simulink model "ES102A_PolarityCfg"  (R2013b)
settings: Solver=ode45  StartTime=0.0  StopTime=10.0  RelTol=1e-3
undefined symbols (not defined in the file): sigbuilder_block
libraries: simulink x29
(part 1 of 4)
settings Model: RequirementInfo={'doors' '00006113' '1' 'false' 'DOORS Surrogate Item' '' } %GIDa_8876c5aa_43e1_47bf_bb90_3f74317f85a0  reqMgrSettings="100 S'doors','misc'{{S'surrogatepath','savemodel','savesurrogate','updateLinks','doorsLinks2sl','slLinks2Doors','purgeDoors','purgeSimulink','detaillevel','surrogateId','synctime'{{T\"/ESG Group/ES102A_PolarityCfg\",M[1],M[1],M[0],M[0],M[0],M[0],M[0],M[1],T\"00006113\",T\"\"}},S'mode','pathStorage'{{T\"generic\",T\"modelRelative\"}}}}"  Creator=pz79n7  LastModifiedBy=NZG49T
settings DataIOCC: SaveFormat=Structure

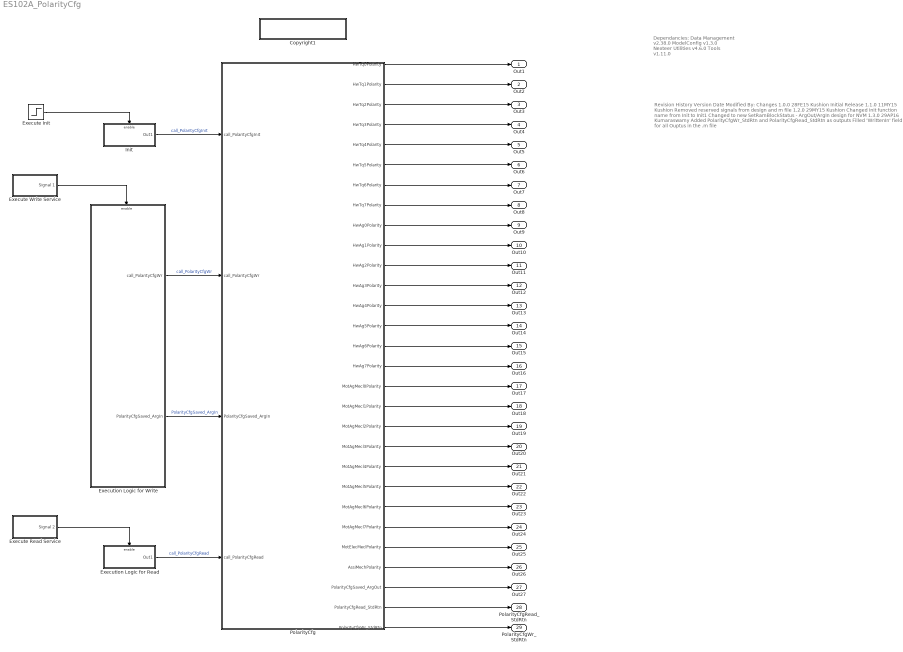
== system ES102A_PolarityCfg ==
  note: Revision History
      |
      | Version		Date 		Modified By: 		Changes
      | 1.0.0 		28FE15		Kushion			Initial Release
      | 1.1.0		11MY15		Kushion			Removed reserved signals from design and m file
      | 1.2.0              29MY15        Kushion			Changed init function name from Init to Init1
      | 										Changed to new SetRamBlockStatus - ArgOut/ArgIn design for NVM
      | 1.3.0		29AP16		Kumaraswamy	Added PolarityCfgWr_StdRtn and PolarityCfgRead_StdRtn as outputs
      | 										Filled 'WrittenIn' field for all Ouptus in the .m file
  note: Dependancies:
      |
      |    Data Management v2.38.0
      |    ModelConfig v1.3.0
      |    Nexteer Utilities v4.6.0
      |    Tools v1.11.0
  Copyright1 : Subsystem  Description=|  mask(Copyright Information){none=on}
      | Copyright info block.                                               
      |                                                                     
      | Place copyright information at the top of every subsystem in design.
      mask prompts: none "No parameters"
      mask help: Place copyright information at the top of every subsystem in design.
      mask Display:
      | NxtrConf = 'Nexteer Confidential';
      | 
      | sys = bdroot; %handle for the current model ("system")
      | first = get_param(sys,'Created');
      | if(isempty(first))
      |     first = datestr(now,'yyyy');
      | else
      |     first = first(end-3:end);  %year is last four digits
      | end
      | 
      | last = get_param(sys,'LastModifiedDate');
      | if isempty(last)
      |     last = datestr(now,'yyyy');
      | else
      |     last = last(end-3:end);
      | end
      | 
      | if strcmp(first,last)
      |     fprintf('%s\nCopyright  %s Nexteer',NxtrConf,first);
      | else
      |     fprintf('%s\n%s%s-%s Nexteer',NxtrConf,char(169),first,last);
      | end
  Execute Init : Step  Time=0.002  Before=1  After=0  SampleTime=0
  Execute Read Service : Subsystem  Tag=STV Subsys  RequirementInfo={} %GIDa_aa5db022_3107_4021_b4bb_b6752dc48d57  LoadFcn=sigbuilder_block('load');  StartFcn=sigbuilder_block('start');  StopFcn=sigbuilder_block('stop');  ClipboardFcn=sigbuilder_block('clipboard');  mask(Sigbuilder block){}
      mask help: Simulink:masks:SigbuilderBlock_MD
      mask init:
      | if ~strcmp(get_param(bdroot(gcbh),'SimulationStatus'),'stopped') tuvar = sigbuilder_block('maskInit'); end
      settings: CopyFcn=sigbuilder_block('copy');  DeleteFcn=sigbuilder_block('delete');  ModelCloseFcn=sigbuilder_block('modelClose');  PreSaveFcn=sigbuilder_block('preSave');  PauseFcn=sigbuilder_block('pause');  ContinueFcn=sigbuilder_block('continue');  NameChangeFcn=sigbuilder_block('namechange');  OpenFcn=sigbuilder_block('open',[437.25 118.5 550.5 394.5 ]);  CloseFcn=sigbuilder_block('close');
      mask Display: plot(0, 0, 100, 100,[2, 2, 32, 32, 2], [68, 8, 8, 68, 68],[32, 2], [38, 38], [32, 19, 2],[53, 60, 44], [32, 17, 17, 2],[16, 16, 31, 31]);txt = getActiveGroup(gcbh);text(2, 100, txt,'verticalAlignment', 'top');
  Execute Write Service : Subsystem  Tag=STV Subsys  RequirementInfo={} %GIDa_7764aa85_78e4_46ff_b91e_6bc780200c88  LoadFcn=sigbuilder_block('load');  StartFcn=sigbuilder_block('start');  StopFcn=sigbuilder_block('stop');  ClipboardFcn=sigbuilder_block('clipboard');  mask(Sigbuilder block){}
      mask help: Simulink:masks:SigbuilderBlock_MD
      mask init:
      | if ~strcmp(get_param(bdroot(gcbh),'SimulationStatus'),'stopped') tuvar = sigbuilder_block('maskInit'); end
      settings: CopyFcn=sigbuilder_block('copy');  DeleteFcn=sigbuilder_block('delete');  ModelCloseFcn=sigbuilder_block('modelClose');  PreSaveFcn=sigbuilder_block('preSave');  PauseFcn=sigbuilder_block('pause');  ContinueFcn=sigbuilder_block('continue');  NameChangeFcn=sigbuilder_block('namechange');  OpenFcn=sigbuilder_block('open',[437.25 118.5 550.5 394.5 ]);  CloseFcn=sigbuilder_block('close');
      mask Display: plot(0, 0, 100, 100,[2, 2, 32, 32, 2], [68, 8, 8, 68, 68],[32, 2], [38, 38], [32, 19, 2],[53, 60, 44], [32, 17, 17, 2],[16, 16, 31, 31]);txt = getActiveGroup(gcbh);text(2, 100, txt,'verticalAlignment', 'top');
  Execution Logic for Read : Subsystem  TreatAsAtomicUnit=on
  Execution Logic for Write : Subsystem  TreatAsAtomicUnit=on
  Init : Subsystem  TreatAsAtomicUnit=on
  PolarityCfg : Subsystem  RequirementInfo={'doors' '00006113' '2' 'false' 'DOORS Surrogate Item' '' } %GIDa_b5b2a4cf_7b68_4330_844c_0f051cc88fcd
      settings: AttributesFormatString=ES102A
  Out1 : Outport
  Out2 : Outport  Port=2
  Out3 : Outport  Port=3
  Out4 : Outport  Port=4
  Out5 : Outport  Port=5
  Out6 : Outport  Port=6
  Out7 : Outport  Port=7
  Out8 : Outport  Port=8
  Out9 : Outport  Port=9
  Out10 : Outport  Port=10
  Out11 : Outport  Port=11
  Out12 : Outport  Port=12
  Out13 : Outport  Port=13
  Out14 : Outport  Port=14
  Out15 : Outport  Port=15
  Out16 : Outport  Port=16
  Out17 : Outport  Port=17
  Out18 : Outport  Port=18
  Out19 : Outport  Port=19
  Out20 : Outport  Port=20
  Out21 : Outport  Port=21
  Out22 : Outport  Port=22
  Out23 : Outport  Port=23
  Out24 : Outport  Port=24
  Out25 : Outport  Port=25
  Out26 : Outport  Port=26
  Out27 : Outport  Port=27
  PolarityCfgRead_StdRtn : Outport  Port=28
  PolarityCfgWr_StdRtn : Outport  Port=29
  wires:
  Init/1(Out1) -> PolarityCfg/1(call_PolarityCfgInit)  "call_PolarityCfgInit"
  Execution Logic for Write/1(call_PolarityCfgWr) -> PolarityCfg/2(call_PolarityCfgWr)  "call_PolarityCfgWr"
  Execute Write Service/1(Signal 1) -> Execution Logic for Write/Enable
  PolarityCfg/1(HwTq0Polarity) -> Out1/1
  PolarityCfg/2(HwTq1Polarity) -> Out2/1
  PolarityCfg/3(HwTq2Polarity) -> Out3/1
  PolarityCfg/4(HwTq3Polarity) -> Out4/1
  PolarityCfg/5(HwTq4Polarity) -> Out5/1
  PolarityCfg/6(HwTq5Polarity) -> Out6/1
  PolarityCfg/7(HwTq6Polarity) -> Out7/1
  PolarityCfg/8(HwTq7Polarity) -> Out8/1
  PolarityCfg/9(HwAg0Polarity) -> Out9/1
  PolarityCfg/10(HwAg1Polarity) -> Out10/1
  PolarityCfg/11(HwAg2Polarity) -> Out11/1
  PolarityCfg/12(HwAg3Polarity) -> Out12/1
  PolarityCfg/13(HwAg4Polarity) -> Out13/1
  PolarityCfg/14(HwAg5Polarity) -> Out14/1
  PolarityCfg/15(HwAg6Polarity) -> Out15/1
  PolarityCfg/16(HwAg7Polarity) -> Out16/1
  PolarityCfg/17(MotAgMecl0Polarity) -> Out17/1
  PolarityCfg/18(MotAgMecl1Polarity) -> Out18/1
  PolarityCfg/19(MotAgMecl2Polarity) -> Out19/1
  PolarityCfg/20(MotAgMecl3Polarity) -> Out20/1
  PolarityCfg/21(MotAgMecl4Polarity) -> Out21/1
  PolarityCfg/22(MotAgMecl5Polarity) -> Out22/1
  PolarityCfg/23(MotAgMecl6Polarity) -> Out23/1
  PolarityCfg/24(MotAgMecl7Polarity) -> Out24/1
  PolarityCfg/25(MotElecMeclPolarity) -> Out25/1
  PolarityCfg/26(AssiMechPolarity) -> Out26/1
  Execute Init/1 -> Init/Enable
  Execution Logic for Read/1(Out1) -> PolarityCfg/4(call_PolarityCfgRead)  "call_PolarityCfgRead"
  Execute Read Service/1(Signal 2) -> Execution Logic for Read/Enable
  Execution Logic for Write/2(PolarityCfgSaved_ArgIn) -> PolarityCfg/3(PolarityCfgSaved_ArgIn)  "PolarityCfgSaved_ArgIn"
  PolarityCfg/27(PolarityCfgSaved_ArgOut) -> Out27/1
  PolarityCfg/29(PolarityCfgWr_StdRtn) -> PolarityCfgWr_StdRtn/1
  PolarityCfg/28(PolarityCfgRead_StdRtn) -> PolarityCfgRead_StdRtn/1

== system ES102A_PolarityCfg/Copyright1 ==

== system ES102A_PolarityCfg/Execute Read Service ==
  Demux : Demux  Tag=STV Demux  Outputs=1
  FromWs : FromWorkspace  Tag=STV FromWs  VariableName=tuvar  SampleTime=0
      SigBuilderData=|
      | common.afterFinalStr = 'Extrapolate'
      | common.sampleTime = 0
      | dataSet.timeRange = [0 10]
      | dataSet.name = 'Group 1'
      | sbobj.Groups.Name = 'Group 1'
      | sbobj.Groups.Signals.Name = 'Signal 2'
      | sbobj.Groups.Signals.XData = [0 5.02 5.02 5.3 5.3 10]
      | sbobj.Groups.Signals.YData = [0 0 1 1 0 0]
  Signal 2 : Outport  Tag=STV Outport
  wires:
  FromWs/1 -> Demux/1
  Demux/1 -> Signal 2/1

== system ES102A_PolarityCfg/Execute Write Service ==
  Demux : Demux  Tag=STV Demux  Outputs=1
  FromWs : FromWorkspace  Tag=STV FromWs  VariableName=tuvar  SampleTime=0
      SigBuilderData=|
      | common.afterFinalStr = 'Extrapolate'
      | common.sampleTime = 0
      | dataSet.timeRange = [0 10]
      | dataSet.name = 'Group 1'
      | sbobj.Groups.Name = 'Group 1'
      | sbobj.Groups.Signals.Name = 'Signal 1'
      | sbobj.Groups.Signals.XData = [0 2.02 2.02 2.12 2.12 10]
      | sbobj.Groups.Signals.YData = [0 0 1 1 0 0]
  Signal 1 : Outport  Tag=STV Outport
  wires:
  Demux/1 -> Signal 1/1
  FromWs/1 -> Demux/1

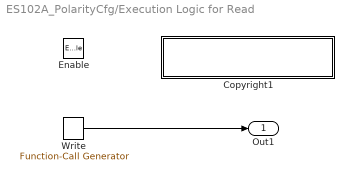
== system ES102A_PolarityCfg/Execution Logic for Read ==
  Enable : EnablePort
  Copyright1 : Subsystem  Description=|  mask(Copyright Information){none=on}
      | Copyright info block.                                               
      |                                                                     
      | Place copyright information at the top of every subsystem in design.
      mask prompts: none "No parameters"
      mask help: Place copyright information at the top of every subsystem in design.
      mask Display:
      | NxtrConf = 'Nexteer Confidential';
      | 
      | sys = bdroot; %handle for the current model ("system")
      | first = get_param(sys,'Created');
      | if(isempty(first))
      |     first = datestr(now,'yyyy');
      | else
      |     first = first(end-3:end);  %year is last four digits
      | end
      | 
      | last = get_param(sys,'LastModifiedDate');
      | if isempty(last)
      |     last = datestr(now,'yyyy');
      | else
      |     last = last(end-3:end);
      | end
      | 
      | if strcmp(first,last)
      |     fprintf('%s\nCopyright  %s Nexteer',NxtrConf,first);
      | else
      |     fprintf('%s\n%s%s-%s Nexteer',NxtrConf,char(169),first,last);
      | end
  "Write " : simulink/Ports & Subsystems/Function-Call Generator  sample_time=0.001  numberOfIterations=1
  Out1 : Outport
  wires:
  "Write "/1 -> Out1/1

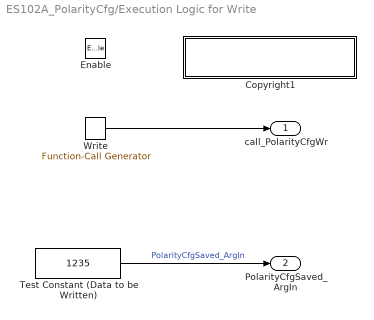
== system ES102A_PolarityCfg/Execution Logic for Write ==
  Enable : EnablePort
  Copyright1 : Subsystem  Description=|  mask(Copyright Information){none=on}
      | Copyright info block.                                               
      |                                                                     
      | Place copyright information at the top of every subsystem in design.
      mask prompts: none "No parameters"
      mask help: Place copyright information at the top of every subsystem in design.
      mask Display:
      | NxtrConf = 'Nexteer Confidential';
      | 
      | sys = bdroot; %handle for the current model ("system")
      | first = get_param(sys,'Created');
      | if(isempty(first))
      |     first = datestr(now,'yyyy');
      | else
      |     first = first(end-3:end);  %year is last four digits
      | end
      | 
      | last = get_param(sys,'LastModifiedDate');
      | if isempty(last)
      |     last = datestr(now,'yyyy');
      | else
      |     last = last(end-3:end);
      | end
      | 
      | if strcmp(first,last)
      |     fprintf('%s\nCopyright  %s Nexteer',NxtrConf,first);
      | else
      |     fprintf('%s\n%s%s-%s Nexteer',NxtrConf,char(169),first,last);
      | end
  Test Constant (Data to be Written) : Constant  Value=1235  OutDataTypeStr=uint32
  "Write " : simulink/Ports & Subsystems/Function-Call Generator  sample_time=0.001  numberOfIterations=1
  call_PolarityCfgWr : Outport
  PolarityCfgSaved_ArgIn : Outport  Port=2
  wires:
  "Write "/1 -> call_PolarityCfgWr/1
  Test Constant (Data to be Written)/1 -> PolarityCfgSaved_ArgIn/1  "PolarityCfgSaved_ArgIn"

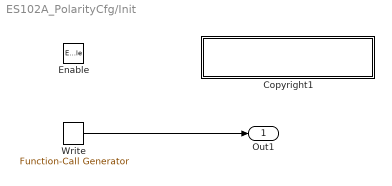
== system ES102A_PolarityCfg/Init ==
  Enable : EnablePort
  Copyright1 : Subsystem  Description=|  mask(Copyright Information){none=on}
      | Copyright info block.                                               
      |                                                                     
      | Place copyright information at the top of every subsystem in design.
      mask prompts: none "No parameters"
      mask help: Place copyright information at the top of every subsystem in design.
      mask Display:
      | NxtrConf = 'Nexteer Confidential';
      | 
      | sys = bdroot; %handle for the current model ("system")
      | first = get_param(sys,'Created');
      | if(isempty(first))
      |     first = datestr(now,'yyyy');
      | else
      |     first = first(end-3:end);  %year is last four digits
      | end
      | 
      | last = get_param(sys,'LastModifiedDate');
      | if isempty(last)
      |     last = datestr(now,'yyyy');
      | else
      |     last = last(end-3:end);
      | end
      | 
      | if strcmp(first,last)
      |     fprintf('%s\nCopyright  %s Nexteer',NxtrConf,first);
      | else
      |     fprintf('%s\n%s%s-%s Nexteer',NxtrConf,char(169),first,last);
      | end
  "Write " : simulink/Ports & Subsystems/Function-Call Generator  sample_time=0.001  numberOfIterations=1
  Out1 : Outport
  wires:
  "Write "/1 -> Out1/1

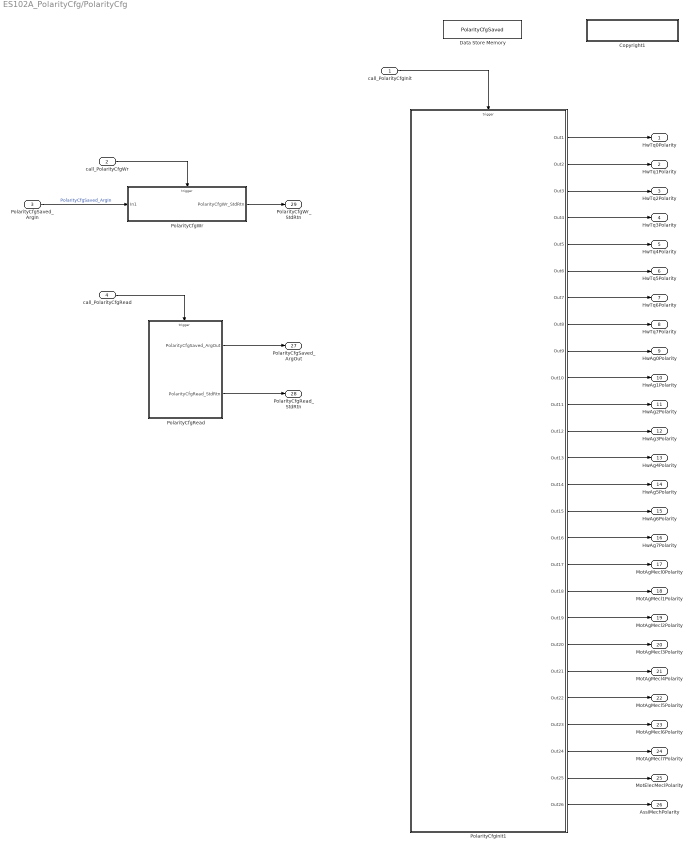
== system ES102A_PolarityCfg/PolarityCfg ==
  call_PolarityCfgInit : Inport  RequirementInfo={'linktype_rmi_doors' '0000c464 (/ESG Group/FDD Module Requirements/EA4 Specific/ES102A_PolarityCfg_Draft)' '#ES102A_77' 'true' 'REQ: ES102A_77' '' } %GIDa_944764bc_0cb2_4aaa_9ac3_90277142e9b4
  call_PolarityCfgWr : Inport  RequirementInfo={'linktype_rmi_doors' '0000c464 (/ESG Group/FDD Module Requirements/EA4 Specific/ES102A_PolarityCfg_Draft)' '#ES102A_77' 'true' 'REQ: ES102A_77' '' } %GIDa_9b084d30_7359_42b6_8a15_ad1a70b28ec8  Port=2
  PolarityCfgSaved_ArgIn : Inport  RequirementInfo={'linktype_rmi_doors' '0000c464 (/ESG Group/FDD Module Requirements/EA4 Specific/ES102A_PolarityCfg_Draft)' '#ES102A_77' 'true' 'REQ: ES102A_77' '' } %GIDa_a6466957_c27f_4df8_8539_2a76a78e8c4a  Port=3
  call_PolarityCfgRead : Inport  RequirementInfo={'linktype_rmi_doors' '0000c464 (/ESG Group/FDD Module Requirements/EA4 Specific/ES102A_PolarityCfg_Draft)' '#ES102A_77' 'true' 'REQ: ES102A_77' '' } %GIDa_531b2b13_38b0_4169_b1e6_83fb34a63da6  Port=4
  Copyright1 : Subsystem  Description=|  mask(Copyright Information){none=on}
      | Copyright info block.                                               
      |                                                                     
      | Place copyright information at the top of every subsystem in design.
      mask prompts: none "No parameters"
      mask help: Place copyright information at the top of every subsystem in design.
      mask Display:
      | NxtrConf = 'Nexteer Confidential';
      | 
      | sys = bdroot; %handle for the current model ("system")
      | first = get_param(sys,'Created');
      | if(isempty(first))
      |     first = datestr(now,'yyyy');
      | else
      |     first = first(end-3:end);  %year is last four digits
      | end
      | 
      | last = get_param(sys,'LastModifiedDate');
      | if isempty(last)
      |     last = datestr(now,'yyyy');
      | else
      |     last = last(end-3:end);
      | end
      | 
      | if strcmp(first,last)
      |     fprintf('%s\nCopyright  %s Nexteer',NxtrConf,first);
      | else
      |     fprintf('%s\n%s%s-%s Nexteer',NxtrConf,char(169),first,last);
      | end
  Data Store Memory : DataStoreMemory  RequirementInfo={'linktype_rmi_doors' '0000c464 (/ESG Group/FDD Module Requirements/EA4 Specific/ES102A_PolarityCfg_Draft)' '#ES102A_121' 'true' 'REQ: ES102A_121' '' } %GIDa_45b83819_743e_4690_820c_6e378aae8028  DataStoreName=PolarityCfgSaved  WriteAfterWriteMsg=warning  WriteAfterReadMsg=warning  InitialValue=128  OutDataTypeStr=uint32  StateMustResolveToSignalObject=on
  PolarityCfgInit1 : Subsystem  RequirementInfo={'doors' '00006113' '4' 'false' 'DOORS Surrogate Item' '' } %GIDa_1863c3af_b51f_4e55_9975_5d17f8ac8b4f  TreatAsAtomicUnit=on
  PolarityCfgRead : Subsystem  RequirementInfo={'linktype_rmi_doors' '0000c464 (/ESG Group/FDD Module Requirements/EA4 Specific/ES102A_PolarityCfg_Draft)' '#ES102A_32' 'true' 'REQ: ES102A_32' '' } %GIDa_7dfc28ec_1f7c_476c_8c67_b6e8513d0710  TreatAsAtomicUnit=on
  PolarityCfgWr : Subsystem  RequirementInfo={'linktype_rmi_doors' '0000c464 (/ESG Group/FDD Module Requirements/EA4 Specific/ES102A_PolarityCfg_Draft)' '#ES102A_123' 'true' 'REQ: ES102A_123' '' } %GIDa_0e7462f6_6bf9_4f9d_a915_7da9c5afb0f4  TreatAsAtomicUnit=on
  HwTq0Polarity : Outport
  HwTq1Polarity : Outport  Port=2
  HwTq2Polarity : Outport  Port=3
  HwTq3Polarity : Outport  Port=4
  HwTq4Polarity : Outport  Port=5
  HwTq5Polarity : Outport  Port=6
  HwTq6Polarity : Outport  Port=7
  HwTq7Polarity : Outport  Port=8
  HwAg0Polarity : Outport  Port=9
  HwAg1Polarity : Outport  Port=10
  HwAg2Polarity : Outport  Port=11
  HwAg3Polarity : Outport  Port=12
  HwAg4Polarity : Outport  Port=13
  HwAg5Polarity : Outport  Port=14
  HwAg6Polarity : Outport  Port=15
  HwAg7Polarity : Outport  Port=16
  MotAgMecl0Polarity : Outport  Port=17
  MotAgMecl1Polarity : Outport  Port=18
  MotAgMecl2Polarity : Outport  Port=19
  MotAgMecl3Polarity : Outport  Port=20
  MotAgMecl4Polarity : Outport  Port=21
  MotAgMecl5Polarity : Outport  Port=22
  MotAgMecl6Polarity : Outport  Port=23
  MotAgMecl7Polarity : Outport  Port=24
  MotElecMeclPolarity : Outport  Port=25
  AssiMechPolarity : Outport  Port=26
  PolarityCfgSaved_ArgOut : Outport  Port=27
  PolarityCfgRead_StdRtn : Outport  Port=28
  PolarityCfgWr_StdRtn : Outport  Port=29
  wires:
  call_PolarityCfgInit/1 -> PolarityCfgInit1/Trigger
  PolarityCfgInit1/1(Out1) -> HwTq0Polarity/1
  PolarityCfgInit1/2(Out2) -> HwTq1Polarity/1
  PolarityCfgInit1/25(Out25) -> MotElecMeclPolarity/1
  PolarityCfgInit1/24(Out24) -> MotAgMecl7Polarity/1
  PolarityCfgInit1/23(Out23) -> MotAgMecl6Polarity/1
  PolarityCfgInit1/22(Out22) -> MotAgMecl5Polarity/1
  PolarityCfgInit1/21(Out21) -> MotAgMecl4Polarity/1
  PolarityCfgInit1/20(Out20) -> MotAgMecl3Polarity/1
  PolarityCfgInit1/19(Out19) -> MotAgMecl2Polarity/1
  PolarityCfgInit1/18(Out18) -> MotAgMecl1Polarity/1
  PolarityCfgInit1/17(Out17) -> MotAgMecl0Polarity/1
  PolarityCfgInit1/16(Out16) -> HwAg7Polarity/1
  PolarityCfgInit1/15(Out15) -> HwAg6Polarity/1
  PolarityCfgInit1/14(Out14) -> HwAg5Polarity/1
  PolarityCfgInit1/13(Out13) -> HwAg4Polarity/1
  PolarityCfgInit1/12(Out12) -> HwAg3Polarity/1
  PolarityCfgInit1/11(Out11) -> HwAg2Polarity/1
  PolarityCfgInit1/10(Out10) -> HwAg1Polarity/1
  PolarityCfgInit1/9(Out9) -> HwAg0Polarity/1
  PolarityCfgInit1/8(Out8) -> HwTq7Polarity/1
  PolarityCfgInit1/7(Out7) -> HwTq6Polarity/1
  PolarityCfgInit1/6(Out6) -> HwTq5Polarity/1
  PolarityCfgInit1/5(Out5) -> HwTq4Polarity/1
  PolarityCfgInit1/4(Out4) -> HwTq3Polarity/1
  PolarityCfgInit1/3(Out3) -> HwTq2Polarity/1
  call_PolarityCfgWr/1 -> PolarityCfgWr/Trigger
  PolarityCfgSaved_ArgIn/1 -> PolarityCfgWr/1(In1)  "PolarityCfgSaved_ArgIn"
  call_PolarityCfgRead/1 -> PolarityCfgRead/Trigger
  PolarityCfgInit1/26(Out26) -> AssiMechPolarity/1
  PolarityCfgRead/1(PolarityCfgSaved_ArgOut) -> PolarityCfgSaved_ArgOut/1
  PolarityCfgRead/2(PolarityCfgRead_StdRtn) -> PolarityCfgRead_StdRtn/1
  PolarityCfgWr/1(PolarityCfgWr_StdRtn) -> PolarityCfgWr_StdRtn/1

== system ES102A_PolarityCfg/Execution Logic for Read/Copyright1 ==

== system ES102A_PolarityCfg/Execution Logic for Write/Copyright1 ==

== system ES102A_PolarityCfg/Init/Copyright1 ==

== system ES102A_PolarityCfg/PolarityCfg/Copyright1 ==

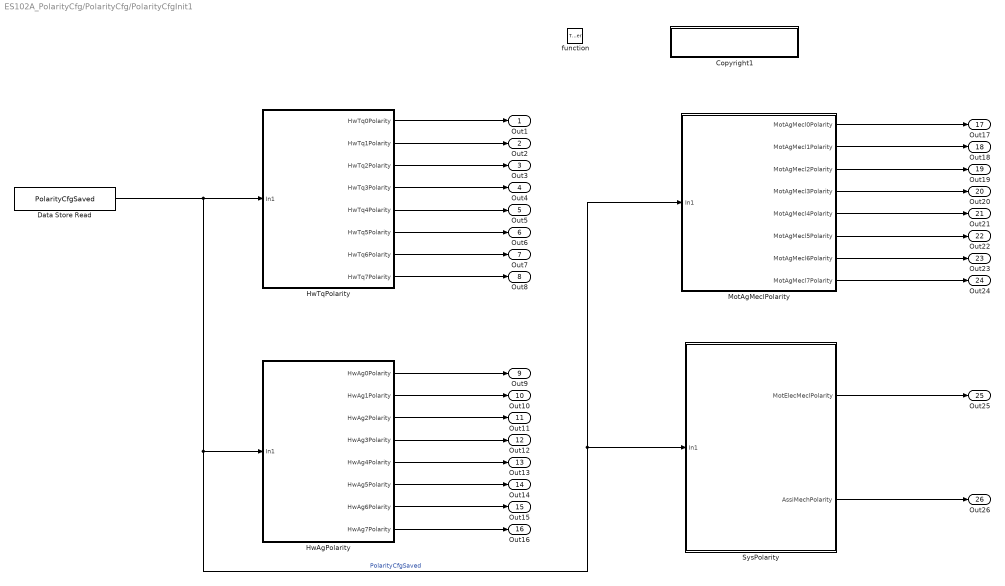
== system ES102A_PolarityCfg/PolarityCfg/PolarityCfgInit1 ==
  function : TriggerPort  TriggerType=function-call
  Copyright1 : Subsystem  Description=|  mask(Copyright Information){none=on}
      | Copyright info block.                                               
      |                                                                     
      | Place copyright information at the top of every subsystem in design.
      mask prompts: none "No parameters"
      mask help: Place copyright information at the top of every subsystem in design.
      mask Display:
      | NxtrConf = 'Nexteer Confidential';
      | 
      | sys = bdroot; %handle for the current model ("system")
      | first = get_param(sys,'Created');
      | if(isempty(first))
      |     first = datestr(now,'yyyy');
      | else
      |     first = first(end-3:end);  %year is last four digits
      | end
      | 
      | last = get_param(sys,'LastModifiedDate');
      | if isempty(last)
      |     last = datestr(now,'yyyy');
      | else
      |     last = last(end-3:end);
      | end
      | 
      | if strcmp(first,last)
      |     fprintf('%s\nCopyright  %s Nexteer',NxtrConf,first);
      | else
      |     fprintf('%s\n%s%s-%s Nexteer',NxtrConf,char(169),first,last);
      | end
  Data Store Read : DataStoreRead  RequirementInfo={'doors' '00006113' '5' 'false' 'DOORS Surrogate Item' '' ; 'linktype_rmi_doors' '0000c464 (/ESG Group/FDD Module Requirements/EA4 Specific/ES102A_PolarityCfg_Draft)' '#ES102A_121' 'true' 'REQ: ES102A_121' '' } %GIDa_907e527e_77c7_4e83_bb56_06805f19a4a8  DataStoreName=PolarityCfgSaved
  HwAgPolarity : Subsystem  RequirementInfo={'doors' '00006113' '6' 'false' 'DOORS Surrogate Item' '' } %GIDa_429eb043_6710_4436_a3ca_3c00e55619f5
  HwTqPolarity : Subsystem  RequirementInfo={'doors' '00006113' '31' 'false' 'DOORS Surrogate Item' '' } %GIDa_bbb4162a_21d1_4e45_9cd3_3deddb2c9dd0
  MotAgMeclPolarity : Subsystem  RequirementInfo={} %GIDa_2cfe3676_9a10_47e9_a295_75323dd5ab14
  SysPolarity : Subsystem  RequirementInfo={'doors' '00006113' '81' 'false' 'DOORS Surrogate Item' '' } %GIDa_7111db3b_6288_48c0_98e0_0710abf9cf17
  Out1 : Outport
  Out2 : Outport  Port=2
  Out3 : Outport  Port=3
  Out4 : Outport  Port=4
  Out5 : Outport  Port=5
  Out6 : Outport  Port=6
  Out7 : Outport  Port=7
  Out8 : Outport  Port=8
  Out9 : Outport  Port=9
  Out10 : Outport  Port=10
  Out11 : Outport  Port=11
  Out12 : Outport  Port=12
  Out13 : Outport  Port=13
  Out14 : Outport  Port=14
  Out15 : Outport  Port=15
  Out16 : Outport  Port=16
  Out17 : Outport  Port=17
  Out18 : Outport  Port=18
  Out19 : Outport  Port=19
  Out20 : Outport  Port=20
  Out21 : Outport  Port=21
  Out22 : Outport  Port=22
  Out23 : Outport  Port=23
  Out24 : Outport  Port=24
  Out25 : Outport  Port=25
  Out26 : Outport  Port=26
  wires:
  HwTqPolarity/1(HwTq0Polarity) -> Out1/1
  Data Store Read/1 -> HwTqPolarity/1(In1), SysPolarity/1(In1), MotAgMeclPolarity/1(In1), HwAgPolarity/1(In1)  "PolarityCfgSaved"
  HwAgPolarity/1(HwAg0Polarity) -> Out9/1
  HwAgPolarity/2(HwAg1Polarity) -> Out10/1
  MotAgMeclPolarity/1(MotAgMecl0Polarity) -> Out17/1
  MotAgMeclPolarity/2(MotAgMecl1Polarity) -> Out18/1
  MotAgMeclPolarity/3(MotAgMecl2Polarity) -> Out19/1
  MotAgMeclPolarity/4(MotAgMecl3Polarity) -> Out20/1
  MotAgMeclPolarity/5(MotAgMecl4Polarity) -> Out21/1
  MotAgMeclPolarity/6(MotAgMecl5Polarity) -> Out22/1
  MotAgMeclPolarity/7(MotAgMecl6Polarity) -> Out23/1
  MotAgMeclPolarity/8(MotAgMecl7Polarity) -> Out24/1
  SysPolarity/1(MotElecMeclPolarity) -> Out25/1
  SysPolarity/2(AssiMechPolarity) -> Out26/1
  HwAgPolarity/3(HwAg2Polarity) -> Out11/1
  HwAgPolarity/4(HwAg3Polarity) -> Out12/1
  HwAgPolarity/5(HwAg4Polarity) -> Out13/1
  HwAgPolarity/6(HwAg5Polarity) -> Out14/1
  HwAgPolarity/7(HwAg6Polarity) -> Out15/1
  HwAgPolarity/8(HwAg7Polarity) -> Out16/1
  HwTqPolarity/2(HwTq1Polarity) -> Out2/1
  HwTqPolarity/3(HwTq2Polarity) -> Out3/1
  HwTqPolarity/4(HwTq3Polarity) -> Out4/1
  HwTqPolarity/5(HwTq4Polarity) -> Out5/1
  HwTqPolarity/6(HwTq5Polarity) -> Out6/1
  HwTqPolarity/7(HwTq6Polarity) -> Out7/1
  HwTqPolarity/8(HwTq7Polarity) -> Out8/1

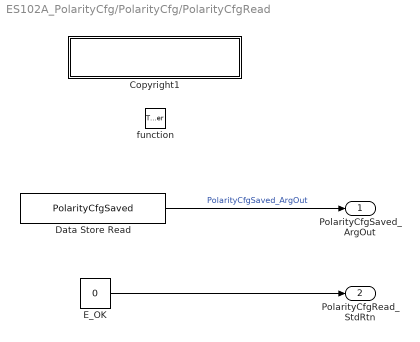
== system ES102A_PolarityCfg/PolarityCfg/PolarityCfgRead ==
  function : TriggerPort  TriggerType=function-call
  Copyright1 : Subsystem  Description=|  mask(Copyright Information){none=on}
      | Copyright info block.                                               
      |                                                                     
      | Place copyright information at the top of every subsystem in design.
      mask prompts: none "No parameters"
      mask help: Place copyright information at the top of every subsystem in design.
      mask Display:
      | NxtrConf = 'Nexteer Confidential';
      | 
      | sys = bdroot; %handle for the current model ("system")
      | first = get_param(sys,'Created');
      | if(isempty(first))
      |     first = datestr(now,'yyyy');
      | else
      |     first = first(end-3:end);  %year is last four digits
      | end
      | 
      | last = get_param(sys,'LastModifiedDate');
      | if isempty(last)
      |     last = datestr(now,'yyyy');
      | else
      |     last = last(end-3:end);
      | end
      | 
      | if strcmp(first,last)
      |     fprintf('%s\nCopyright  %s Nexteer',NxtrConf,first);
      | else
      |     fprintf('%s\n%s%s-%s Nexteer',NxtrConf,char(169),first,last);
      | end
  Data Store Read : DataStoreRead  DataStoreName=PolarityCfgSaved
  E_OK : Constant  Value=0
  PolarityCfgSaved_ArgOut : Outport
  PolarityCfgRead_StdRtn : Outport  Port=2
  wires:
  Data Store Read/1 -> PolarityCfgSaved_ArgOut/1  "PolarityCfgSaved_ArgOut"
  E_OK/1 -> PolarityCfgRead_StdRtn/1

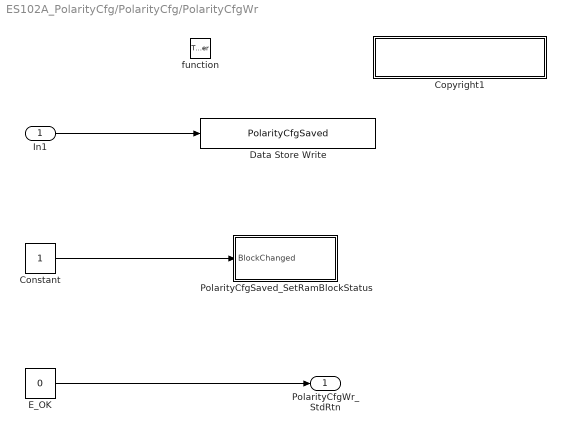
== system ES102A_PolarityCfg/PolarityCfg/PolarityCfgWr ==
  In1 : Inport  OutDataTypeStr=uint32
  function : TriggerPort  TriggerType=function-call
  Constant : Constant
  Copyright1 : Subsystem  Description=|  mask(Copyright Information){none=on}
      | Copyright info block.                                               
      |                                                                     
      | Place copyright information at the top of every subsystem in design.
      mask prompts: none "No parameters"
      mask help: Place copyright information at the top of every subsystem in design.
      mask Display:
      | NxtrConf = 'Nexteer Confidential';
      | 
      | sys = bdroot; %handle for the current model ("system")
      | first = get_param(sys,'Created');
      | if(isempty(first))
      |     first = datestr(now,'yyyy');
      | else
      |     first = first(end-3:end);  %year is last four digits
      | end
      | 
      | last = get_param(sys,'LastModifiedDate');
      | if isempty(last)
      |     last = datestr(now,'yyyy');
      | else
      |     last = last(end-3:end);
      | end
      | 
      | if strcmp(first,last)
      |     fprintf('%s\nCopyright  %s Nexteer',NxtrConf,first);
      | else
      |     fprintf('%s\n%s%s-%s Nexteer',NxtrConf,char(169),first,last);
      | end
  Data Store Write : DataStoreWrite  RequirementInfo={} %GIDa_8506db05_c5df_4358_a563_d10290818754  DataStoreName=PolarityCfgSaved
  E_OK : Constant  Value=0
  PolarityCfgSaved_SetRamBlockStatus : Subsystem
  PolarityCfgWr_StdRtn : Outport
  wires:
  In1/1 -> Data Store Write/1
  Constant/1 -> PolarityCfgSaved_SetRamBlockStatus/1(BlockChanged)
  E_OK/1 -> PolarityCfgWr_StdRtn/1

== system ES102A_PolarityCfg/PolarityCfg/PolarityCfgInit1/Copyright1 ==

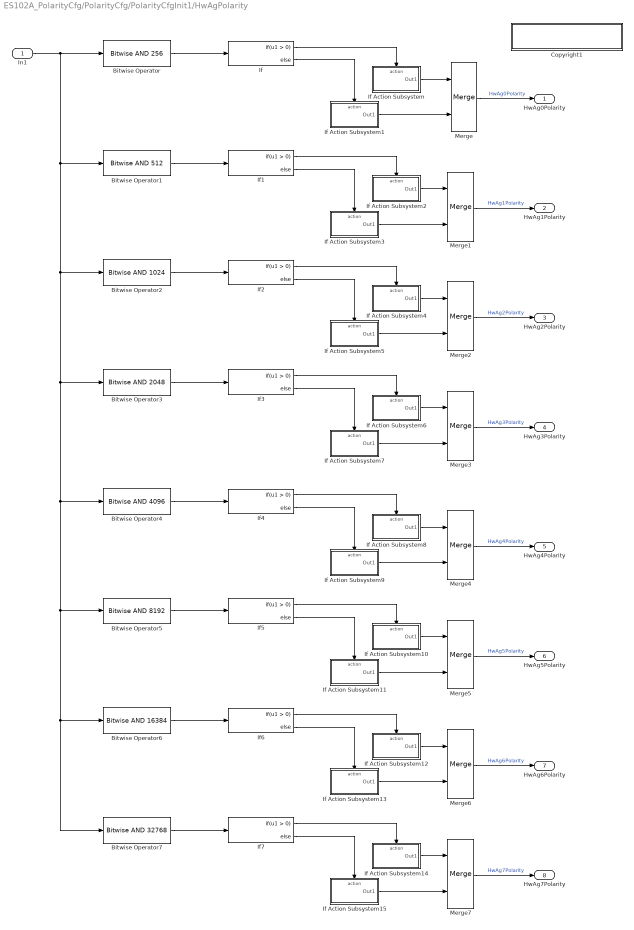
== system ES102A_PolarityCfg/PolarityCfg/PolarityCfgInit1/HwAgPolarity ==
  In1 : Inport
  Bitwise Operator : simulink/Logic and Bit Operations/Bitwise Operator  logicop=AND  UseBitMask=on  BitMask=256  BitMaskRealWorld=Stored Integer
  Bitwise Operator1 : simulink/Logic and Bit Operations/Bitwise Operator  logicop=AND  UseBitMask=on  BitMask=512  BitMaskRealWorld=Stored Integer
  Bitwise Operator2 : simulink/Logic and Bit Operations/Bitwise Operator  logicop=AND  UseBitMask=on  BitMask=1024  BitMaskRealWorld=Stored Integer
  Bitwise Operator3 : simulink/Logic and Bit Operations/Bitwise Operator  logicop=AND  UseBitMask=on  BitMask=2048  BitMaskRealWorld=Stored Integer
  Bitwise Operator4 : simulink/Logic and Bit Operations/Bitwise Operator  logicop=AND  UseBitMask=on  BitMask=4096  BitMaskRealWorld=Stored Integer
  Bitwise Operator5 : simulink/Logic and Bit Operations/Bitwise Operator  logicop=AND  UseBitMask=on  BitMask=8192  BitMaskRealWorld=Stored Integer
  Bitwise Operator6 : simulink/Logic and Bit Operations/Bitwise Operator  logicop=AND  UseBitMask=on  BitMask=16384  BitMaskRealWorld=Stored Integer
  Bitwise Operator7 : simulink/Logic and Bit Operations/Bitwise Operator  logicop=AND  UseBitMask=on  BitMask=32768  BitMaskRealWorld=Stored Integer
  Copyright1 : Subsystem  Description=|  mask(Copyright Information){none=on}
      | Copyright info block.                                               
      |                                                                     
      | Place copyright information at the top of every subsystem in design.
      mask prompts: none "No parameters"
      mask help: Place copyright information at the top of every subsystem in design.
      mask Display:
      | NxtrConf = 'Nexteer Confidential';
      | 
      | sys = bdroot; %handle for the current model ("system")
      | first = get_param(sys,'Created');
      | if(isempty(first))
      |     first = datestr(now,'yyyy');
      | else
      |     first = first(end-3:end);  %year is last four digits
      | end
      | 
      | last = get_param(sys,'LastModifiedDate');
      | if isempty(last)
      |     last = datestr(now,'yyyy');
      | else
      |     last = last(end-3:end);
      | end
      | 
      | if strcmp(first,last)
      |     fprintf('%s\nCopyright  %s Nexteer',NxtrConf,first);
      | else
      |     fprintf('%s\n%s%s-%s Nexteer',NxtrConf,char(169),first,last);
      | end
  If{,1..7} (8 alike) : If
  If Action Subsystem : Subsystem  RequirementInfo={'linktype_rmi_doors' '0000c464 (/ESG Group/FDD Module Requirements/EA4 Specific/ES102A_PolarityCfg_Draft)' '#ES102A_80' 'true' 'REQ: ES102A_80' '' } %GIDa_8ff87bdc_8b23_408f_8f29_411bdc1ae841  TreatAsAtomicUnit=on
  If Action Subsystem1 : Subsystem  RequirementInfo={'linktype_rmi_doors' '0000c464 (/ESG Group/FDD Module Requirements/EA4 Specific/ES102A_PolarityCfg_Draft)' '#ES102A_120' 'true' 'REQ: ES102A_120' '' } %GIDa_6db3e5cb_fe4a_4734_ad38_a4320e3be608  TreatAsAtomicUnit=on
  If Action Subsystem10 : Subsystem  RequirementInfo={'linktype_rmi_doors' '0000c464 (/ESG Group/FDD Module Requirements/EA4 Specific/ES102A_PolarityCfg_Draft)' '#ES102A_80' 'true' 'REQ: ES102A_80' '' } %GIDa_94c95c94_4a65_4260_91bb_98fda14128f8  TreatAsAtomicUnit=on
  If Action Subsystem11 : Subsystem  RequirementInfo={'linktype_rmi_doors' '0000c464 (/ESG Group/FDD Module Requirements/EA4 Specific/ES102A_PolarityCfg_Draft)' '#ES102A_120' 'true' 'REQ: ES102A_120' '' } %GIDa_af8c3124_da6f_456f_a4a1_ef06d1c336ef  TreatAsAtomicUnit=on
  If Action Subsystem12 : Subsystem  RequirementInfo={'linktype_rmi_doors' '0000c464 (/ESG Group/FDD Module Requirements/EA4 Specific/ES102A_PolarityCfg_Draft)' '#ES102A_80' 'true' 'REQ: ES102A_80' '' } %GIDa_f31c3091_3bd1_4157_8595_6b84c9a53787  TreatAsAtomicUnit=on
  If Action Subsystem13 : Subsystem  RequirementInfo={'linktype_rmi_doors' '0000c464 (/ESG Group/FDD Module Requirements/EA4 Specific/ES102A_PolarityCfg_Draft)' '#ES102A_120' 'true' 'REQ: ES102A_120' '' } %GIDa_1a124141_9c5c_4a14_a626_5b29274fc7ee  TreatAsAtomicUnit=on
  If Action Subsystem14 : Subsystem  RequirementInfo={'linktype_rmi_doors' '0000c464 (/ESG Group/FDD Module Requirements/EA4 Specific/ES102A_PolarityCfg_Draft)' '#ES102A_80' 'true' 'REQ: ES102A_80' '' } %GIDa_ac1fbc5b_82cb_4db7_aa7a_7c2f80c7b7f5  TreatAsAtomicUnit=on
  If Action Subsystem15 : Subsystem  RequirementInfo={'linktype_rmi_doors' '0000c464 (/ESG Group/FDD Module Requirements/EA4 Specific/ES102A_PolarityCfg_Draft)' '#ES102A_120' 'true' 'REQ: ES102A_120' '' } %GIDa_fa056db4_cfe4_4461_8c09_b84af17e0b79  TreatAsAtomicUnit=on
  If Action Subsystem2 : Subsystem  RequirementInfo={'linktype_rmi_doors' '0000c464 (/ESG Group/FDD Module Requirements/EA4 Specific/ES102A_PolarityCfg_Draft)' '#ES102A_80' 'true' 'REQ: ES102A_80' '' } %GIDa_a8ee91d0_e47c_4f28_abaa_44643e1e807b  TreatAsAtomicUnit=on
  If Action Subsystem3 : Subsystem  RequirementInfo={'linktype_rmi_doors' '0000c464 (/ESG Group/FDD Module Requirements/EA4 Specific/ES102A_PolarityCfg_Draft)' '#ES102A_120' 'true' 'REQ: ES102A_120' '' } %GIDa_5041c8f2_8441_4859_8481_2f6e90bf806c  TreatAsAtomicUnit=on
  If Action Subsystem4 : Subsystem  RequirementInfo={'linktype_rmi_doors' '0000c464 (/ESG Group/FDD Module Requirements/EA4 Specific/ES102A_PolarityCfg_Draft)' '#ES102A_80' 'true' 'REQ: ES102A_80' '' } %GIDa_805988a0_51d6_4213_8ad1_6e581be5a356  TreatAsAtomicUnit=on
  If Action Subsystem5 : Subsystem  RequirementInfo={'linktype_rmi_doors' '0000c464 (/ESG Group/FDD Module Requirements/EA4 Specific/ES102A_PolarityCfg_Draft)' '#ES102A_120' 'true' 'REQ: ES102A_120' '' } %GIDa_9b43575c_c923_43ef_833a_6b67eba0aff7  TreatAsAtomicUnit=on
  If Action Subsystem6 : Subsystem  RequirementInfo={'linktype_rmi_doors' '0000c464 (/ESG Group/FDD Module Requirements/EA4 Specific/ES102A_PolarityCfg_Draft)' '#ES102A_80' 'true' 'REQ: ES102A_80' '' } %GIDa_770aa32a_ac6f_42ee_8ef3_2c06b5267f4c  TreatAsAtomicUnit=on
  If Action Subsystem7 : Subsystem  RequirementInfo={'linktype_rmi_doors' '0000c464 (/ESG Group/FDD Module Requirements/EA4 Specific/ES102A_PolarityCfg_Draft)' '#ES102A_120' 'true' 'REQ: ES102A_120' '' } %GIDa_3f5aa05c_b40c_4514_9dec_59bfcd0105a4  TreatAsAtomicUnit=on
  If Action Subsystem8 : Subsystem  RequirementInfo={'linktype_rmi_doors' '0000c464 (/ESG Group/FDD Module Requirements/EA4 Specific/ES102A_PolarityCfg_Draft)' '#ES102A_80' 'true' 'REQ: ES102A_80' '' } %GIDa_aa96187a_ca5d_440e_9c8c_3b5a2b216bc9  TreatAsAtomicUnit=on
  If Action Subsystem9 : Subsystem  RequirementInfo={'linktype_rmi_doors' '0000c464 (/ESG Group/FDD Module Requirements/EA4 Specific/ES102A_PolarityCfg_Draft)' '#ES102A_120' 'true' 'REQ: ES102A_120' '' } %GIDa_4b7b4bb4_7ded_4f81_b48e_6052cb6669fb  TreatAsAtomicUnit=on
  Merge : Merge  RequirementInfo={'linktype_rmi_doors' '0000c464 (/ESG Group/FDD Module Requirements/EA4 Specific/ES102A_PolarityCfg_Draft)' '#ES102A_103' 'true' 'REQ: ES102A_103' '' } %GIDa_59a7a3cb_7337_4b31_818a_32558171d388
  Merge1 : Merge  RequirementInfo={'linktype_rmi_doors' '0000c464 (/ESG Group/FDD Module Requirements/EA4 Specific/ES102A_PolarityCfg_Draft)' '#ES102A_104' 'true' 'REQ: ES102A_104' '' } %GIDa_fdcfb2ce_1b23_455c_93b3_933620cb3305
  Merge2 : Merge  RequirementInfo={'linktype_rmi_doors' '0000c464 (/ESG Group/FDD Module Requirements/EA4 Specific/ES102A_PolarityCfg_Draft)' '#ES102A_105' 'true' 'REQ: ES102A_105' '' } %GIDa_a2bb3062_d161_4046_91dc_eca7623ba778
  Merge3 : Merge  RequirementInfo={'linktype_rmi_doors' '0000c464 (/ESG Group/FDD Module Requirements/EA4 Specific/ES102A_PolarityCfg_Draft)' '#ES102A_106' 'true' 'REQ: ES102A_106' '' } %GIDa_00cf674c_357f_4672_a266_54b9d11d602d
  Merge4 : Merge  RequirementInfo={'linktype_rmi_doors' '0000c464 (/ESG Group/FDD Module Requirements/EA4 Specific/ES102A_PolarityCfg_Draft)' '#ES102A_107' 'true' 'REQ: ES102A_107' '' } %GIDa_fd8725ba_8ed7_4008_9db9_7fdf568da15e
  Merge5 : Merge  RequirementInfo={'linktype_rmi_doors' '0000c464 (/ESG Group/FDD Module Requirements/EA4 Specific/ES102A_PolarityCfg_Draft)' '#ES102A_108' 'true' 'REQ: ES102A_108' '' } %GIDa_2e80fb71_3a47_4594_a693_48606176cc57
  Merge6 : Merge  RequirementInfo={'linktype_rmi_doors' '0000c464 (/ESG Group/FDD Module Requirements/EA4 Specific/ES102A_PolarityCfg_Draft)' '#ES102A_109' 'true' 'REQ: ES102A_109' '' } %GIDa_8917b656_8f4f_4904_b9a7_46da1e2e9a4f
  Merge7 : Merge  RequirementInfo={'linktype_rmi_doors' '0000c464 (/ESG Group/FDD Module Requirements/EA4 Specific/ES102A_PolarityCfg_Draft)' '#ES102A_110' 'true' 'REQ: ES102A_110' '' } %GIDa_7f0f22da_03c7_4863_b236_93f47e4bb252
  HwAg0Polarity : Outport  RequirementInfo={'doors' '00006113' '23' 'false' 'DOORS Surrogate Item' '' ; 'linktype_rmi_doors' '0000c464 (/ESG Group/FDD Module Requirements/EA4 Specific/ES102A_PolarityCfg_Draft)' '#ES102A_103' 'true' 'REQ: ES102A_103' '' } %GIDa_f1a26782_1215_48ac_8d50_f9c7d349a7f2
  HwAg1Polarity : Outport  RequirementInfo={'doors' '00006113' '24' 'false' 'DOORS Surrogate Item' '' ; 'linktype_rmi_doors' '0000c464 (/ESG Group/FDD Module Requirements/EA4 Specific/ES102A_PolarityCfg_Draft)' '#ES102A_104' 'true' 'REQ: ES102A_104' '' } %GIDa_dd376297_0365_4bbd_9d50_249b8ed8a650  Port=2
  HwAg2Polarity : Outport  RequirementInfo={'doors' '00006113' '25' 'false' 'DOORS Surrogate Item' '' ; 'linktype_rmi_doors' '0000c464 (/ESG Group/FDD Module Requirements/EA4 Specific/ES102A_PolarityCfg_Draft)' '#ES102A_105' 'true' 'REQ: ES102A_105' '' } %GIDa_8f12dca0_8fe0_43c3_a152_8c81b9de991f  Port=3
  HwAg3Polarity : Outport  RequirementInfo={'doors' '00006113' '26' 'false' 'DOORS Surrogate Item' '' ; 'linktype_rmi_doors' '0000c464 (/ESG Group/FDD Module Requirements/EA4 Specific/ES102A_PolarityCfg_Draft)' '#ES102A_106' 'true' 'REQ: ES102A_106' '' } %GIDa_2072d969_7886_4a6f_ac7d_d21fec6a4fd9  Port=4
  HwAg4Polarity : Outport  RequirementInfo={'doors' '00006113' '27' 'false' 'DOORS Surrogate Item' '' ; 'linktype_rmi_doors' '0000c464 (/ESG Group/FDD Module Requirements/EA4 Specific/ES102A_PolarityCfg_Draft)' '#ES102A_107' 'true' 'REQ: ES102A_107' '' } %GIDa_e0e4c591_18a3_4d32_ba0b_8cff6ecf9793  Port=5
  HwAg5Polarity : Outport  RequirementInfo={'doors' '00006113' '28' 'false' 'DOORS Surrogate Item' '' ; 'linktype_rmi_doors' '0000c464 (/ESG Group/FDD Module Requirements/EA4 Specific/ES102A_PolarityCfg_Draft)' '#ES102A_108' 'true' 'REQ: ES102A_108' '' } %GIDa_59102869_db34_456e_a087_fa6f2d9be894  Port=6
  HwAg6Polarity : Outport  RequirementInfo={'doors' '00006113' '29' 'false' 'DOORS Surrogate Item' '' ; 'linktype_rmi_doors' '0000c464 (/ESG Group/FDD Module Requirements/EA4 Specific/ES102A_PolarityCfg_Draft)' '#ES102A_109' 'true' 'REQ: ES102A_109' '' } %GIDa_4c4f5277_9cf6_4e74_95f0_34e3ee28be35  Port=7
  HwAg7Polarity : Outport  RequirementInfo={'doors' '00006113' '30' 'false' 'DOORS Surrogate Item' '' ; 'linktype_rmi_doors' '0000c464 (/ESG Group/FDD Module Requirements/EA4 Specific/ES102A_PolarityCfg_Draft)' '#ES102A_110' 'true' 'REQ: ES102A_110' '' } %GIDa_b4280782_f714_4d39_9585_862fa3d8d8f2  Port=8
  wires:
  Bitwise Operator/1 -> If/1
  If/1 -> If Action Subsystem/Action
  If/2 -> If Action Subsystem1/Action
  If Action Subsystem/1(Out1) -> Merge/1
  If Action Subsystem1/1(Out1) -> Merge/2
  Merge/1 -> HwAg0Polarity/1  "HwAg0Polarity"
  Bitwise Operator1/1 -> If1/1
  If1/1 -> If Action Subsystem2/Action
  If1/2 -> If Action Subsystem3/Action
  If Action Subsystem2/1(Out1) -> Merge1/1
  If Action Subsystem3/1(Out1) -> Merge1/2
  Merge1/1 -> HwAg1Polarity/1  "HwAg1Polarity"
  Bitwise Operator2/1 -> If2/1
  If2/1 -> If Action Subsystem4/Action
  If2/2 -> If Action Subsystem5/Action
  If Action Subsystem4/1(Out1) -> Merge2/1
  If Action Subsystem5/1(Out1) -> Merge2/2
  Merge2/1 -> HwAg2Polarity/1  "HwAg2Polarity"
  Bitwise Operator3/1 -> If3/1
  If3/1 -> If Action Subsystem6/Action
  If3/2 -> If Action Subsystem7/Action
  If Action Subsystem6/1(Out1) -> Merge3/1
  If Action Subsystem7/1(Out1) -> Merge3/2
  Merge3/1 -> HwAg3Polarity/1  "HwAg3Polarity"
  Bitwise Operator4/1 -> If4/1
  If4/1 -> If Action Subsystem8/Action
  If4/2 -> If Action Subsystem9/Action
  If Action Subsystem8/1(Out1) -> Merge4/1
  If Action Subsystem9/1(Out1) -> Merge4/2
  Merge4/1 -> HwAg4Polarity/1  "HwAg4Polarity"
  Bitwise Operator5/1 -> If5/1
  If5/1 -> If Action Subsystem10/Action
  If5/2 -> If Action Subsystem11/Action
  If Action Subsystem10/1(Out1) -> Merge5/1
  If Action Subsystem11/1(Out1) -> Merge5/2
  Merge5/1 -> HwAg5Polarity/1  "HwAg5Polarity"
  In1/1 -> Bitwise Operator2/1, Bitwise Operator6/1, Bitwise Operator7/1, Bitwise Operator5/1, Bitwise Operator4/1, Bitwise Operator3/1, Bitwise Operator1/1, Bitwise Operator/1
  Bitwise Operator6/1 -> If6/1
  If6/1 -> If Action Subsystem12/Action
  If6/2 -> If Action Subsystem13/Action
  If Action Subsystem12/1(Out1) -> Merge6/1
  If Action Subsystem13/1(Out1) -> Merge6/2
  Merge6/1 -> HwAg6Polarity/1  "HwAg6Polarity"
  Bitwise Operator7/1 -> If7/1
  If7/1 -> If Action Subsystem14/Action
  If7/2 -> If Action Subsystem15/Action
  If Action Subsystem14/1(Out1) -> Merge7/1
  If Action Subsystem15/1(Out1) -> Merge7/2
  Merge7/1 -> HwAg7Polarity/1  "HwAg7Polarity"
